simulink model "phase_lead"  (Simulink 6.4)
settings: Solver=FixedStepDiscrete  StartTime=0.0  StopTime=10.0  RelTol=1e-3
settings Model: LastModifiedBy=Gordon

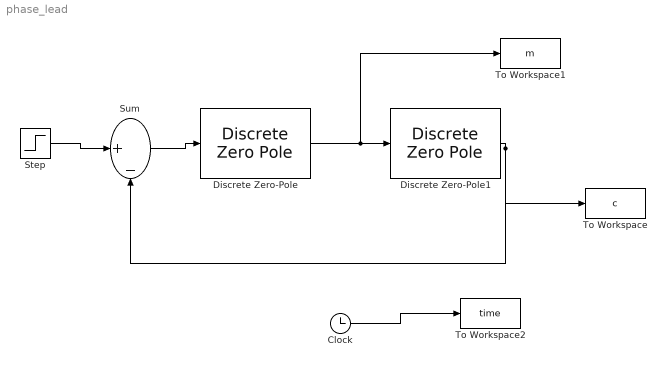
== system phase_lead ==
  Clock : Clock
      settings: Decimation=10
  Discrete Zero-Pole : DiscreteZeroPole  Zeros=[0.4]  Poles=[-1]  Gain=0.104  SampleTime=0.8
  Discrete Zero-Pole1 : DiscreteZeroPole  Zeros=[]  Poles=[1 0.5]  Gain=10  SampleTime=0.8
  Step : Step  Time=0.8  SampleTime=0.8
  Sum : Sum  Inputs=|+-
  To Workspace : ToWorkspace  VariableName=c  SampleTime=0.8  SaveFormat=Array
  To Workspace1 : ToWorkspace  VariableName=m  SampleTime=0.8  SaveFormat=Array
  To Workspace2 : ToWorkspace  VariableName=time  SampleTime=0.8  SaveFormat=Array
  wires:
  Sum/1 -> Discrete Zero-Pole/1
  Discrete Zero-Pole1/1 -> Sum/2, To Workspace/1
  Discrete Zero-Pole/1 -> Discrete Zero-Pole1/1, To Workspace1/1
  Step/1 -> Sum/1
  Clock/1 -> To Workspace2/1
